simulink library "ilcPathOpt_cl"  (R2018b)
settings: Solver=VariableStepAuto  StartTime=0.0  StopTime=10.0  RelTol=1e-3
undefined symbols (not defined in the file or in its folder): hiLvlCtrl, initializeBussesFromBlock
libraries: firstOrderFilter_ul x1, ilcPerfIndx_cl x1, ilcPhase_cl x1, ilcUpdate_cl x1
settings Model: Creator=mcobb  LastModifiedBy=mcobb

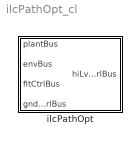
== system ilcPathOpt_cl ==
  ilcPathOpt : Subsystem  LoadFcn=initializeBussesFromBlock(gcb)  InitFcn=initializeBussesFromBlock(gcb)  StartFcn=initializeBussesFromBlock(gcb)  mask{ctrl=hiLvlCtrl}
      mask prompts: ctrl "Controller Object"

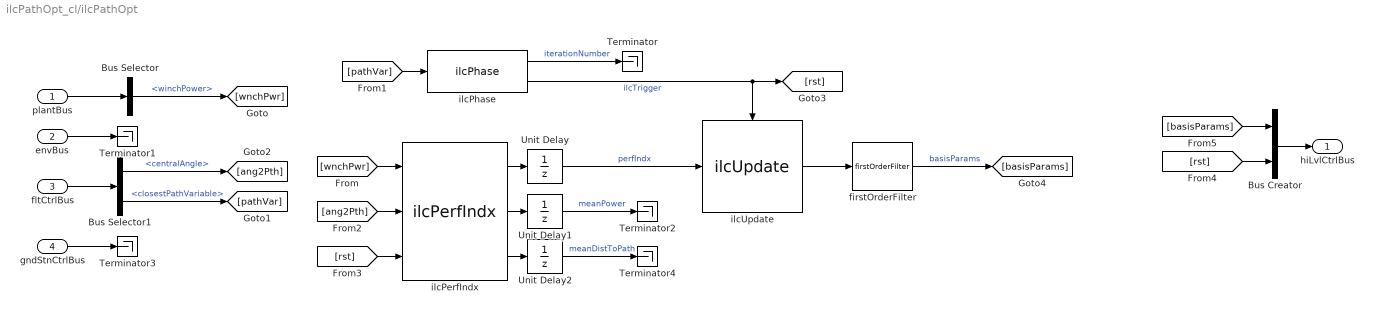
== system ilcPathOpt_cl/ilcPathOpt ==
  plantBus : Inport  OutDataTypeStr=Bus: plantBus
  envBus : Inport  Port=2  OutDataTypeStr=Bus: envBus
  fltCtrlBus : Inport  Port=3  OutDataTypeStr=Bus: fltCtrlBus
  gndStnCtrlBus : Inport  Port=4  OutDataTypeStr=Bus: gndStnCtrlBus
  Bus Creator : BusCreator  Inputs=2  OutDataTypeStr=Bus: hiLvlCtrlBus
  Bus Selector : BusSelector  OutputSignals=winchPower
  Bus Selector1 : BusSelector  OutputSignals=centralAngle,closestPathVariable
  Terminator{,1..4} (5 alike) : Terminator
  Unit Delay : UnitDelay  SampleTime=-1
  Unit Delay1 : UnitDelay  SampleTime=-1
  Unit Delay2 : UnitDelay  SampleTime=-1
  firstOrderFilter : firstOrderFilter_ul/firstOrderFilter  tau=ctrl.filtTimeConst.Value  ic=ctrl.initBasisParams.Value
  ilcPerfIndx : ilcPerfIndx_cl/ilcPerfIndx  w=ctrl.distPenaltyWght.Value
  ilcPhase : ilcPhase_cl/ilcPhase  upperLim=ctrl.pathVarUpperLim.Value  lowerLim=ctrl.pathVarLowerLim.Value  numInitLaps=ctrl.numInitLaps.Value
  ilcUpdate : ilcUpdate_cl/ilcUpdate  initBasisParams=ctrl.initBasisParams.Value  lrn=ctrl.learningGain.Value  AdaptationParameter=ctrl.forgettingFactor.Value  trstRgn=ctrl.trustRegion.Value  amp=ctrl.excitationAmp.Value  enableVec=ctrl.optEnable.Value
  hiLvlCtrlBus : Outport  OutDataTypeStr=Bus: hiLvlCtrlBus
  wires:
  Unit Delay/1 -> ilcUpdate/1  "perfIndx"
  plantBus/1 -> Bus Selector/1
  envBus/1 -> Terminator1/1
  fltCtrlBus/1 -> Bus Selector1/1
  gndStnCtrlBus/1 -> Terminator3/1
  Bus Creator/1 -> hiLvlCtrlBus/1
  firstOrderFilter/1 -> [basisParams]  "basisParams"
  Bus Selector/1 -> [wnchPwr]  "<winchPower>"
  [wnchPwr] -> ilcPerfIndx/1
  Bus Selector1/1 -> [ang2Pth]  "<centralAngle>"
  Bus Selector1/2 -> [pathVar]  "<closestPathVariable>"
  [pathVar] -> ilcPhase/1
  [ang2Pth] -> ilcPerfIndx/2
  [rst] -> ilcPerfIndx/3
  ilcPhase/2 -> [rst], ilcUpdate/Trigger  "ilcTrigger"
  ilcPerfIndx/1 -> Unit Delay/1
  ilcUpdate/1 -> firstOrderFilter/1
  ilcPhase/1 -> Terminator/1  "iterationNumber"
  ilcPerfIndx/2 -> Unit Delay1/1
  Unit Delay1/1 -> Terminator2/1  "meanPower"
  Unit Delay2/1 -> Terminator4/1  "meanDistToPath"
  ilcPerfIndx/3 -> Unit Delay2/1
  [rst] -> Bus Creator/2
  [basisParams] -> Bus Creator/1
